simulink library "AvgModels"  (R2015a)
settings: Solver=ode45  StartTime=0.0  StopTime=10.0  RelTol=1e-3
libraries: simulink x12, AvgModels x8
(part 1 of 2)
settings Model: CovSFcnEnable=off  Creator=Luigi Galotto Junior  LastModifiedBy=lgalo
settings DataIOCC: SignalLoggingSaveFormat=ModelDataLogs
settings OptimizationCC: InitFltsAndDblsToZero=on
settings DebuggingCC: SaveWithParameterizedLinksMsg=none  UnderspecifiedInitializationDetection=Classic  MergeDetectMultiDrivingBlocksExec=none  SignalResolutionControl=TryResolveAllWithWarning  SolverPrmCheckMsg=warning  MultiTaskDSMMsg=warning  MultiTaskCondExecSysMsg=none  StrictBusMsg=None
settings GRTTargetCC: TargetFcnLib=ansi_tfl_tmw.mat  CombineOutputUpdateFcns=off  GRTInterface=on

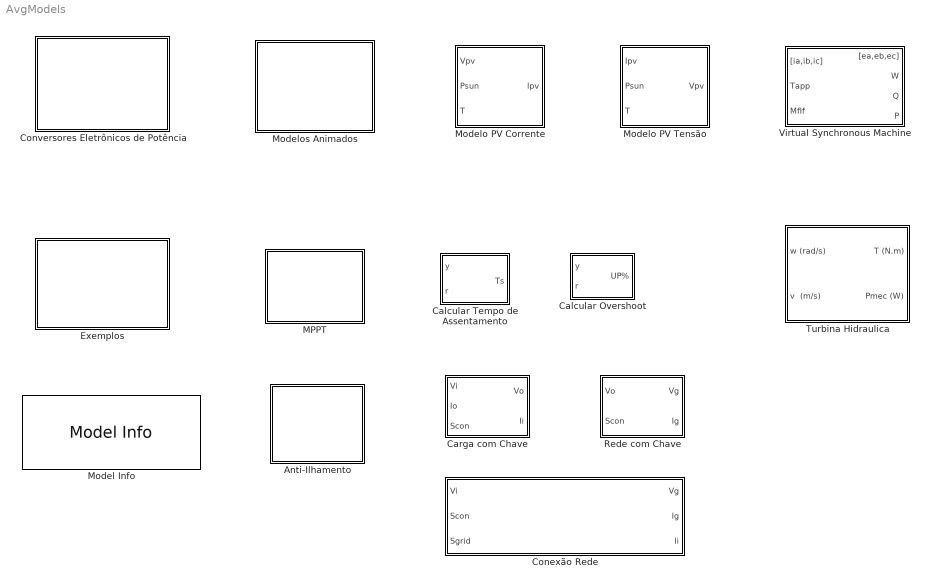
== system AvgModels ==
  Anti-Ilhamento : Subsystem
  Calcular Overshoot : Subsystem  mask(Calc_Up){}
      mask help: Bloco para calcular a Ultrapassagem percentual (UP%) a partir da referência (r) e da resposta da saída (y) no tempo.
  Calcular Tempo de Assentamento : Subsystem  mask(Calc_Ts){}
      mask help: Bloco para calcular o Tempo de Assentamento (Ts), em segundos, a partir da referência (r) e da resposta da saída (y) no tempo.
  Carga com Chave : Subsystem  mask(Modelo Médio de Conexao com a Rede){Rl=100, Rsmin=0.1, Rsmax=1e6}
      mask prompts: Rl "Carga (ohms)"; Rsmin "Resistência on do Relé"; Rsmax "Resistência off do Relé"
      mask help:
      | Simula a conexão de uma fonte de tensão com determinada impedância
      | em uma rede elétrica.
      mask Display:
      | theta = 0:0.1:2*pi;
      | % fundo
      | patch([-1.2 0.3 0.3 -1.2],[-0.1 -0.1 1 1],[1 1 1])
      | 
      | % ------------- circuito da conexao  --------------
      | % circuito
      | plot([-0.9 -0.9 -0.4],[0.1 0.9 0.9])
      | plot([-0.4 -0.3],[0.9 1]) % chave
      | plot([-0.25 0 0],[0.9 0.9 0.1])
      | 
      | % fonte
      | x = 0.15*cos(theta)-0.9;
      | y = 0.15*sin(theta)+0.5;
      | patch(x,y,[1 0.5 0.5]);
      | text(-0.95,0.5,'Vi')
      | 
      | % carga
      | patch([-0.1 0.1 0.1 -0.1],[0.3 0.3 0.6 0.6],[0.5 0.5 1])
      | text(-0.1,0.45,'Rl')
      | 
      | % GND
      | plot([0.80 1]-0.9,[0.1 0.1])
      | plot([0.84 0.96]-0.9,[0.05 0.05])
      | plot([0.88 0.92]-0.9,[0 0]);
      | 
      | plot([0.80 1]-1.8,[0.1 0.1])
      | plot([0.84 0.96]-1.8,[0.05 0.05])
      | plot([0.88 0.92]-1.8,[0 0]);
      | 
      | 
      | % portas
      | port_label('input',1,'Vi')
      | port_label('input',2,'Io')
      | port_label('input',3,'Scon')
      | 
      | port_label('output',1,'Vo')
      | port_label('output',2,'Ii')
  Conexão Rede : Subsystem  mask(Modelo Médio de Conexao com a Rede){Lg=1e-3, Rg=1e-3, Vrede=127, frede=60, Rl=100, Rsmin=0.1, Rsmax=1e6}
      mask prompts: Lg "Indutância da Rede (H)"; Rg "Resistência da Rede (Ohms)"; Vrede "Tensão eficaz da Rede (V)"; frede "Frequência da Rede (Hz)"; Rl "Carga na Rede"; Rsmin "Resistência on do Relé"; Rsmax "Resistência off do Relé"
      mask help:
      | Simula a conexão de uma fonte de tensão com determinada impedância
      | em uma rede elétrica.
      mask Display:
      | theta = 0:0.1:2*pi;
      | % fundo
      | patch([-1.3 1.3 1.3 -1.3],[-0.1 -0.1 1 1],[1 1 1])
      | 
      | % ------------- circuito da conexao  --------------
      | % circuito
      | plot([-0.9 -0.9 -0.4],[0.1 0.9 0.9])
      | plot([-0.4 -0.3],[0.9 1]) % chave
      | plot([-0.25 0 0],[0.9 0.9 0.1])
      | 
      | % fonte
      | x = 0.15*cos(theta)-0.9;
      | y = 0.15*sin(theta)+0.5;
      | patch(x,y,[1 0.5 0.5]);
      | text(-0.95,0.5,'Vi')
      | 
      | % carga
      | patch([-0.1 0.1 0.1 -0.1],[0.3 0.3 0.6 0.6],[0.5 0.5 1])
      | text(-0.05,0.45,'Rl')
      | 
      | % GND
      | plot([0.80 1]-0.9,[0.1 0.1])
      | plot([0.84 0.96]-0.9,[0.05 0.05])
      | plot([0.88 0.92]-0.9,[0 0]);
      | 
      | plot([0.80 1]-1.8,[0.1 0.1])
      | plot([0.84 0.96]-1.8,[0.05 0.05])
      | plot([0.88 0.92]-1.8,[0 0]);
      | 
      | % --------------- circuito da rede -------------
      | % circuito
      | plot([0 0.25],[0.9 0.9])
      | plot([0.3 0.4 0.9 0.9],[1 0.9 0.9 0.1])
      | 
      | % GND
      | plot([0.80 1],[0.1 0.1])
      | plot([0.84 0.96],[0.05 0.05])
      | plot([0.88 0.92],[0 0]);
      | 
      | % controle da chave
      | % plot([0 0.28 0.28],[0.2 0.2 0.9]);
      | 
      | % rede
      | x = 0.15*cos(theta)+0.9;
      | y = 0.15*sin(theta)+0.5;
      | patch(x,y,[1 0.5 0.5])
      | text(0.85,0.5,'Vg')
      | 
      | patch([0.5 0.8 0.8 0.5],[0.8 0.8 1 1],[0.5 0.5 1])
      | text(0.55,0.9,'Zg')
      | 
      | % Texto das chaves
      | text(-0.4,0.7,'Scon')
      | text(0.2,0.7,'Sgrid')
      | 
      | port_label('output',1,'Vg');
      | port_label('output',2,'Ig');
      | port_label('output',2,'Ii');
      | 
      | port_label('input',1,'Vi');
      | port_label('input',2,'Scon');
      | port_label('input',3,'Sgrid');
  Conversores Eletrônicos de Potência : Subsystem
  Exemplos : Subsystem
  MPPT : Subsystem
  Model Info : simulink/Model-Wide Utilities/Model Info  Frame=on  DisplayStringWithTags=|  HorizontalTextAlignment=Center  LeftAlignmentValue=0.5  SourceBlockDiagram=AvgModels  TagMaxNumber=20
      | Conjunto de Blocos de 
      | Modelos Dinâmicos.
      | %<Creator>
      | %<Created>
  Modelo PV Corrente : Subsystem  mask(Modelo PV de corrente){Ms=1, Mp=1, Ns=54, Voc=0.6093, Isc=8.21, Tr=273 + 25, tau=1e-2, Rs=0.005, Rp=7, a=3.18e-3, n=1.2, k=1.38e-23, q=1.60e-19, EG=1.1}
      mask prompts: Ms "Módulos em Série"; Mp "Módulos em Paralelo"; Ns "Número de células"; Voc "Tensão de circuito aberto (Voc por célula)"; Isc "Corrente de curto-circuito (Isc)"; Tr "Temperatura Ambiente (K)"; tau "Constante de Tempo (s)"; Rs "Resistência série"; Rp "Resistência paralela"
      mask help:
      | Este é um modelo de corrente para painéis fotovoltaicos (sozinhos ou em arranjo).
      |
      | Fornece a corrrente esperada de acordo com a tensão, a densidade de potência do sol e a temperatura ambiente.
      |
      | V(PV) é a tensão do arranjo fotovoltaico em volts.
      | Psun é a densidade de potência do sol em W/m2.
      | T é a temperatura ambiente em ºC.
      mask Display:
      | % desenho detalhado
      | patch([0 .5 1 .5],[0 1 1 0],[0 0 1]);
      | plot([0 0.5],[0 1])
      | plot([0.5/3 0.5+0.5/3],[0 1])
      | plot([0.5/3 0.5+0.5/3]+0.5/3,[0 1])
      | plot([0.5 1],[0 1])
      | 
      | plot([0 0.5],[0 0])
      | plot([0 0.5]+0.125,[0 0]+0.25)
      | plot([0 0.5]+0.25,[0 0]+0.5)
      | plot([0 0.5]+0.25+0.125,[0 0]+0.75)
      | plot([0.5 1],[1 1])
      | 
      | 
      | port_label('output',1,'I(PV)');
      | 
      | port_label('input',1,'V(PV)');
      | port_label('input',2,'Psun');
      | port_label('input',3,'T');
  Modelo PV Tensão : Subsystem  mask(Modelo PV de tensão){Ns=54, Voc=0.6093, Isc=8.21, Rs=0.005, Rp=7, Ms=1, Mp=1, Tr=273 + 25, a=3.18e-3, n=1.2, k=1.38e-23, q=1.60e-19, EG=1.1, tau=1e-2, Psun=1000, Animar=on}
      mask prompts: Ns "Número de células"; Voc "Tensão de circuito aberto (Voc por célula)"; Isc "Corrente de curto-circuito (Isc)"; Rs "Resistência série da célula"; Rp "Resistência paralela da célula"; Ms "Módulos em Série"; Mp "Módulos em Paralelo"; Tr "Temperatura Ambiente (K)"; a "Coeficiente de temperatura de Isc:"; n "Fator de qualidade da junção p-n:"; k "Constante de Boltzmann:"; q "Carga do elétron:"; EG "Energia da banda proibida:"; tau "Contante de tempo (s):"; Psun "Irradiação de teste (W/m2):"; Animar "Animar em execução?"
      mask help:
      | Este é um modelo de tensão para painéis fotovoltaicos (sozinhos ou em arranjo).
      |
      | Fornece a tensão esperada de acordo com a corrente, a densidade de potência do sol e a temperatura ambiente.
      |
      | I(PV) é a corrente do arranjo fotovoltaico em Amperes.
      | Psun é a densidade de potência do sol em W/m2.
      | T é a temperatura ambiente em ºC.
      |
      | V(PV) é a tensão do arranjo fotovoltaico em Amperes.
      mask DialogControl Container9 Prompt: Verificação da curva.
      mask DialogControl Control2 Prompt: Verificar Curvas
      mask DialogControl Control2 Callback:
      | Psun = str2num(get_param(gcbh,'Psun'));
      | Tr = str2num(get_param(gcbh,'Tr'));
      | Voc = str2num(get_param(gcbh,'Voc'));
      | Isc = str2num(get_param(gcbh,'Isc'));
      | Rp = str2num(get_param(gcbh,'Rp'));
      | Rs = str2num(get_param(gcbh,'Rs'));
      | Ns = str2num(get_param(gcbh,'Ns'));
      | alpha = str2num(get_param(gcbh,'a'));
      | encontrapmax(Psun,Tr-273,Voc,Isc,Rp,Rs,Ns,alpha);
      mask Display:
      | % desenho detalhado
      | patch([0 .5 1 .5],[0 1 1 0],[0 0 1]);
      | plot([0 0.5],[0 1])
      | plot([0.5/3 0.5+0.5/3],[0 1])
      | plot([0.5/3 0.5+0.5/3]+0.5/3,[0 1])
      | plot([0.5 1],[0 1])
      | 
      | plot([0 0.5],[0 0])
      | plot([0 0.5]+0.125,[0 0]+0.25)
      | plot([0 0.5]+0.25,[0 0]+0.5)
      | plot([0 0.5]+0.25+0.125,[0 0]+0.75)
      | plot([0.5 1],[1 1])
      | 
      | 
      | port_label('output',1,'V(PV)');
      | 
      | port_label('input',1,'I(PV)');
      | port_label('input',2,'Psun');
      | port_label('input',3,'T');
  Modelos Animados : Subsystem
  Rede com Chave : Subsystem  mask(Modelo Médio de Conexao com a Rede){Lg=1e-3, Rg=1e-3, Vrede=127, frede=60, Rsmin=0.1, Rsmax=1e6}
      mask prompts: Lg "Indutância da Rede (H)"; Rg "Resistência da Rede (Ohms)"; Vrede "Tensão eficaz da Rede (V)"; frede "Frequência da Rede (Hz)"; Rsmin "Resistência on do Relé"; Rsmax "Resistência off do Relé"
      mask help:
      | Simula a conexão de uma fonte de tensão em uma rede elétrica
      | com determinada impedância.
      mask Display:
      | theta = 0:0.1:2*pi;
      | % fundo
      | patch([-0.3 1.3 1.3 -0.3],[-0.1 -0.1 1 1],[1 1 1])
      | 
      | % --------------- circuito da rede -------------
      | % circuito
      | plot([0 0.25],[0.9 0.9])
      | plot([0.3 0.4 0.9 0.9],[1 0.9 0.9 0.1])
      | 
      | % GND
      | plot([0.80 1],[0.1 0.1])
      | plot([0.84 0.96],[0.05 0.05])
      | plot([0.88 0.92],[0 0]);
      | 
      | % controle da chave
      | % plot([0 0.28 0.28],[0.2 0.2 0.9]);
      | 
      | % rede
      | x = 0.15*cos(theta)+0.9;
      | y = 0.15*sin(theta)+0.5;
      | patch(x,y,[1 0.5 0.5])
      | text(0.85,0.5,'Vg')
      | 
      | patch([0.5 0.8 0.8 0.5],[0.8 0.8 1 1],[0.5 0.5 1])
      | text(0.55,0.9,'Zg')
      | 
      | 
      | port_label('output',1,'Vg');
      | port_label('output',2,'Ig');
      | 
      | port_label('input',1,'Vi');
      | port_label('input',2,'Scon');
  Turbina Hidraulica : Subsystem  mask(Turbina Pelton){ro=997, Area_bico=(1/4)*pi*0.012^2, gate=Interno (fixo), abertura=1, raio_turbina=0.105, tipo=Pelton, poly=[-0.3915 -0.669 1.52 0.005209]}
      mask prompts: ro "Densidade do fluido (kg/m3)"; Area_bico "Área de entrada do fluido"; gate "Controle do Gate"; abertura "Abertura do Gate (0 a 1)"; raio_turbina "Raio da Turbina"; tipo "Tipos de Turbinas:"; poly "Curva Cp x lambda (polinomio)"
      mask help:
      | Modelo da turbina Pelton em R.P. desenvolvida inicialmente durante
      | o mestrado do acadêmico Júlio Lescano, a partir de dados de um
      | protótipo e de resultados experimentais.
      mask TypeOptions gate: Interno (fixo) | Externo
      mask Callback gate:
      | gate = get_param(gcbh,'gate');
      | p = Simulink.Mask.get(gcb);
      | a = p.Parameters(4);
      | switch gate
      |     case 'Externo'
      |         % a.set('Enable', 'off');
      |     otherwise
      |         % a.set('Enable', 'true');
      | 
      | end
      mask TypeOptions tipo: Pelton | Savonius | Savonius com duto
      mask Callback tipo:
      | tipo = get_param(gcbh,'tipo');
      | switch tipo
      |     case 'Pelton'
      |         set_param(gcbh,'poly','[-0.3915 -0.669 1.52 0.005209]');
      |     case 'Savonius'
      |         set_param(gcbh,'poly','[-0.8682    1.3133   -0.3584]');
      |     case 'Savonius com duto'
      |         set_param(gcbh,'poly','[-0.8682    1.2786   -0.2225]');
      | end
      mask DialogControl Control2 Prompt: Plotar Curvas
      mask DialogControl Control2 Callback:
      | poly = str2num(get_param(gcbh,'poly'));
      | tsr = linspace(0,2,50);
      | plot(tsr,max(polyval(poly,tsr),0))
      | grid;
      | xlabel('\lambda (TSR - Tip Speed Ratio)')
      | ylabel('C_p')
  Virtual Synchronous Machine : Subsystem  mask(Virtual Synchronous Machine (VSM)){J=1e-2, Dpm=1e-4, w0=0}
      mask prompts: J "Inércia:"; Dpm "Atrito Dinâmico:"; w0 "Velocidade Inicial:"
      mask help:
      | Modelo de máquina síncrona virtual (VSM) desenvolvido durante o trabalho de conclusão de curso da aluna Isabela Assis.
      |
      | Objetivo inicial: controlar um inversor emulando uma máquina síncrona, chamado de synchronverter.
      |
      | Também pode ser utilizado como modelo simplificado de máquinas síncronas.

== system AvgModels/Anti-Ilhamento ==
  anti-islanding AFD : Subsystem  mask(Anti-ilhamento AFD){ffalha=62, Df=10}
      mask prompts: ffalha "Frequência de Falha (Hz)"; Df "Variação de frequência (Hz)"
      mask help:
      | Bloco que realiza método ativo de anti-ilhamento AFD (Active Frequency Drift).
      |
      | Pode ser utilizado em conjunto com PLL.
  anti-islanding HF impedance : Subsystem  mask(Anti-ilhamento impedância.){vsinal=2, fsinal=600, vmax=350}
      mask prompts: vsinal "Tensão do Sinal (V)"; fsinal "Frequência do Sinal (Hz)"; vmax "Tensão máxima de detecção (V)"
      mask help:
      | Bloco que realiza método ativo de anti-ilhamento de impedância em alta frequência.
      |
      | Pode ser utilizado em conjunto com PLL.
  anti-islanding SMS : Subsystem  mask(Anti-Ilhamento SMS){fnom=60, fmax=63, angmax=10}
      mask prompts: fnom "Frequência Nominal (Hz)"; fmax "Frequência Máxima (Hz)"; angmax "Ângulo Máximo (graus)"
      mask help:
      | Bloco que realiza método ativo de anti-ilhamento SMS (Sliding Mode Frequency Shift).
      |
      | Pode ser utilizado em conjunto com PLL.

== system AvgModels/Calcular Overshoot ==
  y : Inport
  r : Inport  Port=2
  Difference : simulink/Discrete/Difference  ICPrevInput=0.0  InputProcessing=Inherited  OutMin=[]  OutMax=[]  OutDataType=fixdt(1, 16)  OutScaling=2^-10  DoSatur=off
  Divide : Product  Inputs=*/
  Gain1 : Gain  Gain=100
  Memory : Memory
  Memory1 : Memory
  MinMax : MinMax  Function=max
  MinMax2 : MinMax  Function=max
  Mux1 : Mux  Inputs=2
  Mux2 : Mux  Inputs=2
  Subtract : Sum  Inputs=+-
  amplitude : Display
  UP% : Outport
  wires:
  Memory/1 -> Mux1/2
  Subtract/1 -> Mux1/1
  y/1 -> Subtract/1
  Gain1/1 -> UP%/1
  MinMax/1 -> Divide/1, Memory/1
  Mux1/1 -> MinMax/1
  r/1 -> Difference/1
  Divide/1 -> Gain1/1
  MinMax2/1 -> Memory1/1, amplitude/1, Subtract/2, Divide/2
  Memory1/1 -> Mux2/2
  Difference/1 -> Mux2/1
  Mux2/1 -> MinMax2/1

== system AvgModels/Calcular Tempo de Assentamento ==
  y : Inport
  r : Inport  Port=2
  Abs : Abs
  Compare To Constant : simulink/Logic and Bit Operations/Compare To Constant  relop=>=  const=0.01  OutDataTypeStr=boolean
  Compare To Constant1 : simulink/Logic and Bit Operations/Compare To Constant  relop=>=  const=0.01  OutDataTypeStr=boolean
  Data Type Conversion : DataTypeConversion
  Integrator Limited : Integrator  ExternalReset=falling  LimitOutput=on  LowerSaturationLimit=0
  Logical Operator : Logic  AllPortsSameDT=off
  Sum1 : Sum  Inputs=|+-
  Ts : Outport
  wires:
  Sum1/1 -> Abs/1
  y/1 -> Compare To Constant/1, Integrator Limited/2, Sum1/1
  Integrator Limited/1 -> Ts/1
  Compare To Constant/1 -> Logical Operator/2
  r/1 -> Sum1/2
  Compare To Constant1/1 -> Logical Operator/1
  Data Type Conversion/1 -> Integrator Limited/1
  Abs/1 -> Compare To Constant1/1
  Logical Operator/1 -> Data Type Conversion/1

== system AvgModels/Carga com Chave ==
  Vi : Inport
  Io : Inport  Port=2
  Scon : Inport  Port=3
  Add1 : Sum  Inputs=|+-
  Add2 : Sum  Inputs=|++
  Add3 : Sum  Inputs=|++
  Constant : Constant  Value=Rl
  Product : Product  Inputs=**/
  Product1 : Product
  Product2 : Product  Inputs=*/
  Relay : Relay  OnSwitchValue=0.6  OffSwitchValue=0.4  OnOutputValue=Rsmin  OffOutputValue=Rsmax
  Vo : Outport
  Ii : Outport  Port=2
  wires:
  Product/1 -> Product2/1, Vo/1
  Add2/1 -> Product/3
  Relay/1 -> Add2/2, Product1/2
  Constant/1 -> Product2/2, Product/2, Add2/1
  Scon/1 -> Relay/1
  Vi/1 -> Add1/1
  Io/1 -> Product1/1, Add3/2
  Product1/1 -> Add1/2
  Add1/1 -> Product/1
  Product2/1 -> Add3/1
  Add3/1 -> Ii/1

== system AvgModels/Conexão Rede ==
  Vi : Inport
  Scon : Inport  Port=2
  Sgrid : Inport  Port=3
  Carga com Chave : AvgModels/Carga com Chave  Rl=Rl  Rsmin=Rsmin  Rsmax=Rsmax
  Rede com Chave : AvgModels/Rede com Chave  Lg=Lg  Rg=Rg  Vrede=Vrede  frede=frede  Rsmin=Rsmin  Rsmax=Rsmax
  Vg : Outport
  Ig : Outport  Port=2
  Ii : Outport  Port=3
  wires:
  Carga com Chave/1 -> Rede com Chave/1
  Rede com Chave/1 -> Vg/1
  Rede com Chave/2 -> Carga com Chave/2, Ig/1
  Carga com Chave/2 -> Ii/1
  Vi/1 -> Carga com Chave/1
  Scon/1 -> Carga com Chave/3
  Sgrid/1 -> Rede com Chave/2

== system AvgModels/Conversores Eletrônicos de Potência ==
  Boost : Subsystem  mask(Boost){L=1e-4, RL=0, C=1e-3, Edit_carga=100, Vini=0, Iini=0, Fs=20000, Vdon=0.7, Rdon=0, Vson=0, Rdson=0}
      mask prompts: L "Indutância (H):"; RL "Resistência do Indutor (Ohms):"; C "Capacitância (F):"; Edit_carga "Carga no Capacitor (Ohms):"; Vini "Tensão do Capacitor (V):"; Iini "Corrente do Indutor (A):"; Fs "Frequência de Chaveamento (Hz)"; Vdon "Tensão direta no diodo (V)"; Rdon "Resistência Interna no Diodo"; Vson "Tensão direta na chave (V)"; Rdson "Resistência da Chave"
      mask help:
      | Este bloco modela o comportamento dinâmico médio do conversor CC/CC boost.
      |
      | Este modelo é valido para os modos de condução contínua e descontínua.
      |
      | Quando escolhida a opção (Carga Fixa) a entrada I_out não é utilizada.
      |
      | Desenvolvido por:
      | Luigi Galotto Junior - 21/10/2004
      | Melhorado em 28/09/2017
      mask Display:
      | %image(imread('Boost.jpg'));
      | 
      | % desenho basico
      | %plot([0 1],[0 1])
      | %text(0.3,0.6,'DC')
      | %text(0.6,0.4,'DC')
      | 
      | % desenho detalhado
      | plot([0.0 0.6 0.60 0.5],...
      |      [0.9 0.9 0.60 0.4]);
      | 
      | plot([0 0.6 0.6 0.6 1.1 0.8 0.8 1.1],...
      |      [0 0.0 0.3 0.0 0 0.0 0.9 0.9]);
      | 
      | plot([0.6 0.65 0.65 0.75 0.75 0.75 0.8],...
      |      [0.9 0.90 1.00 0.90 1.00 0.90 0.9])
      | plot([0.6 0.65 0.65 0.75 0.75 0.75 0.8],...
      |      [0.9 0.90 0.80 0.90 0.80 0.90 0.9])
      | 
      | patch([0.25 .5 .5 .25],[0.8 0.8 0.95 0.95],[0 0 1]);
      | patch([0.75 .85 .85 .75],[0.32 0.32 0.6 0.6],[1 0 0]);
      | 
      | text(0.35,0.65,'RL')
      | text(0.65,0.45,'C')
      | 
      | 
      | port_label('output',1,'I in');
      | port_label('output',2,'V out');
      | port_label('input',1,'V in');
      | port_label('input',2,'I out');
      | port_label('input',3,'D');
  Buck : Subsystem  mask(Buck){C=1e-3, L=1e-4, RL=0, Edit_carga=100, Vini=0, Iini=0, Fs=20000, Rdson=10e-3, Vson=0, Rdon=1e-3, Vdon=0.8}
      mask prompts: C "Capacitância (F):"; L "Indutância (H):"; RL "Resistência no Indutor (Ohms):"; Edit_carga "Carga no Capacitor (Ohms)"; Vini "Tensão Inicial do Capacitor (V):"; Iini "Corrente Inicial do Indutor (A):"; Fs "Frequência de Chaveamento (Hz)"; Rdson "Chave (R On)"; Vson "Chave (V On)"; Rdon "Diodo (R On)"; Vdon "Diodo (V On)"
      mask help:
      | Este bloco modela o comportamento dinâmico médio do conversor BUCK CC/CC.
      |
      | Este modelo é valido para os modos de condução contínua e descontínua.
      |
      | Quando escolhida a opção (Carga Fixa) a entrada I_out não é utilizada.
      |
      | Desenvolvido por:
      | Luigi Galotto Junior - 01/10/2017
      mask Display:
      | %image(imread('Boost.jpg'));
      | 
      | % desenho basico
      | plot([0 1],[0 1])
      | text(0.3,0.6,'DC')
      | text(0.6,0.4,'DC')
      | 
      | % desenho detalhado
      | %plot([0.0 0.6 0.60 0.5],...
      | %     [0.9 0.9 0.60 0.4]);
      | 
      | %plot([0 0.6 0.6 0.6 1.1 0.8 0.8 1.1],...
      | %     [0 0.0 0.3 0.0 0 0.0 0.9 0.9]);
      | 
      | %plot([0.6 0.65 0.65 0.75 0.75 0.75 0.8],...
      | %    [0.9 0.90 1.00 0.90 1.00 0.90 0.9])
      | %plot([0.6 0.65 0.65 0.75 0.75 0.75 0.8],...
      | %     [0.9 0.90 0.80 0.90 0.80 0.90 0.9])
      | 
      | %patch([0.25 .5 .5 .25],[0.8 0.8 0.95 0.95],[0 0 1]);
      | %patch([0.75 .85 .85 .75],[0.32 0.32 0.6 0.6],[1 0 0]);
      | 
      | %text(0.35,0.65,'RL')
      | %text(0.65,0.45,'C')
      | 
      | 
      | port_label('output',1,'I in');
      | port_label('output',2,'V out');
      | port_label('input',1,'V in');
      | port_label('input',2,'I out');
      | port_label('input',3,'D');
  Buck-Boost : Subsystem  mask(Buck-Boost){C=1e-3, L=1e-4, RL=0, Edit_carga=100, Vini=0, Iini=0, Fs=20000, Rdson=0, Vson=0, Rdon=0, Vdon=0.8}
      mask prompts: C "Capacitância (F):"; L "Indutância (H):"; RL "Resistência do Indutor (Ohms):"; Edit_carga "Carga no Capacitor (Ohms):"; Vini "Tensão Inicial do Capacitor (V):"; Iini "Corrente Inicial do Indutor (A):"; Fs "Frequência de Chaveamento (Hz)"; Rdson "Chave (R On):"; Vson "Chave (V On):"; Rdon "Diodo (R On):"; Vdon "Diodo (V On):"
      mask help:
      | Este bloco modela o comportamento dinâmico médio do conversor BUCK-BOOST CC/CC.
      |
      | Este modelo é valido para os modos de condução contínua e descontínua.
      |
      | Quando escolhida a opção (Carga Fixa) a entrada I_out não é utilizada.
      |
      | Desenvolvido por:
      | Luigi Galotto Junior - 01/10/2017
      mask Display:
      | %image(imread('Boost.jpg'));
      | 
      | % desenho basico
      | plot([0 1],[0 1])
      | text(0.3,0.6,'DC')
      | text(0.6,0.4,'DC')
      | 
      | % desenho detalhado
      | %plot([0.0 0.6 0.60 0.5],...
      | %     [0.9 0.9 0.60 0.4]);
      | 
      | %plot([0 0.6 0.6 0.6 1.1 0.8 0.8 1.1],...
      | %     [0 0.0 0.3 0.0 0 0.0 0.9 0.9]);
      | 
      | %plot([0.6 0.65 0.65 0.75 0.75 0.75 0.8],...
      | %    [0.9 0.90 1.00 0.90 1.00 0.90 0.9])
      | %plot([0.6 0.65 0.65 0.75 0.75 0.75 0.8],...
      | %     [0.9 0.90 0.80 0.90 0.80 0.90 0.9])
      | 
      | %patch([0.25 .5 .5 .25],[0.8 0.8 0.95 0.95],[0 0 1]);
      | %patch([0.75 .85 .85 .75],[0.32 0.32 0.6 0.6],[1 0 0]);
      | 
      | %text(0.35,0.65,'RL')
      | %text(0.65,0.45,'C')
      | 
      | 
      | port_label('output',1,'I in');
      | port_label('output',2,'V out');
      | port_label('input',1,'V in');
      | port_label('input',2,'I out');
      | port_label('input',3,'D');
  Inversor Boost TriState : Subsystem  mask(Inversor Boost Tri-State){Lb=10e-6, Co=1e-6, ILb=0, Vco=0}
      mask prompts: Lb "Indutância (H)"; Co "Capacitância (F)"; ILb "Corrente do Indutor"; Vco "Tensão no Capacitor"
      mask help:
      | Modelo médio do Inversor Boost Tri-State Integrado.
      |
      | A polaridade da saída é comandada pelo valor de D2 que pode ser positivo ou negativo. O valor máximo de D2 deve ser limitado a 1-D1.
      mask DialogControl Container3 Prompt: Condições Iniciais
      mask Display:
      | %image(imread('Boost.jpg'));
      | 
      | % desenho basico
      | plot([0 1],[0 1])
      | text(0.3,0.6,'DC')
      | text(0.6,0.4,'AC')
      | 
      | % desenho detalhado
      | %plot([0.0 0.6 0.60 0.5],...
      | %     [0.9 0.9 0.60 0.4]);
      | 
      | %plot([0 0.6 0.6 0.6 1.1 0.8 0.8 1.1],...
      | %     [0 0.0 0.3 0.0 0 0.0 0.9 0.9]);
      | 
      | %plot([0.6 0.65 0.65 0.75 0.75 0.75 0.8],...
      | %    [0.9 0.90 1.00 0.90 1.00 0.90 0.9])
      | %plot([0.6 0.65 0.65 0.75 0.75 0.75 0.8],...
      | %     [0.9 0.90 0.80 0.90 0.80 0.90 0.9])
      | 
      | %patch([0.25 .5 .5 .25],[0.8 0.8 0.95 0.95],[0 0 1]);
      | %patch([0.75 .85 .85 .75],[0.32 0.32 0.6 0.6],[1 0 0]);
      | 
      | %text(0.35,0.65,'RL')
      | %text(0.65,0.45,'C')
      | 
      | 
      | port_label('output',1,'I in');
      | port_label('output',2,'V out');
      | port_label('output',3,'I Lin');
      | 
      | port_label('input',1,'V in');
      | port_label('input',2,'I out');
      | port_label('input',3,'D1');
      | port_label('input',4,'D2');
  Inversor Buck-Boost TriState : Subsystem  mask(Inversor Buck-Boost Tri-State){Lb=10e-6, Co=1e-6, ILb=0, Vco=0}
      mask prompts: Lb "Indutância (H)"; Co "Capacitância (F)"; ILb "Corrente do Indutor"; Vco "Tensão no Capacitor"
      mask help:
      | Modelo médio do Inversor Buck-Boost Tri-State Integrado.
      |
      | A polaridade da saída é comandada pelo valor de D2 que pode ser positivo ou negativo. O valor máximo de D2 deve ser limitado a 1-D1.
      mask DialogControl Container3 Prompt: Condições Iniciais
      mask Display:
      | %image(imread('Boost.jpg'));
      | 
      | % desenho basico
      | plot([0 1],[0 1])
      | text(0.3,0.6,'DC')
      | text(0.6,0.4,'AC')
      | 
      | % desenho detalhado
      | %plot([0.0 0.6 0.60 0.5],...
      | %     [0.9 0.9 0.60 0.4]);
      | 
      | %plot([0 0.6 0.6 0.6 1.1 0.8 0.8 1.1],...
      | %     [0 0.0 0.3 0.0 0 0.0 0.9 0.9]);
      | 
      | %plot([0.6 0.65 0.65 0.75 0.75 0.75 0.8],...
      | %    [0.9 0.90 1.00 0.90 1.00 0.90 0.9])
      | %plot([0.6 0.65 0.65 0.75 0.75 0.75 0.8],...
      | %     [0.9 0.90 0.80 0.90 0.80 0.90 0.9])
      | 
      | %patch([0.25 .5 .5 .25],[0.8 0.8 0.95 0.95],[0 0 1]);
      | %patch([0.75 .85 .85 .75],[0.32 0.32 0.6 0.6],[1 0 0]);
      | 
      | %text(0.35,0.65,'RL')
      | %text(0.65,0.45,'C')
      | 
      | 
      | port_label('output',1,'I in');
      | port_label('output',2,'V out');
      | port_label('output',3,'I Lin');
      | 
      | port_label('input',1,'V in');
      | port_label('input',2,'I out');
      | port_label('input',3,'D1');
      | port_label('input',4,'D2');
  Inversor VSI : Subsystem  mask(Inversor Fonte de Tensão (VSI)){Lb=10e-6, Rl=0, Co=1e-6, ILb=0, Vco=0}
      mask prompts: Lb "Indutância do Filtro (H)"; Rl "Resistência do Indutor (Ohms)"; Co "Capacitância do Filtro (F)"; ILb "Corrente do Indutor (A)"; Vco "Tensão no Capacitor (V)"
      mask help:
      | Modelo médio do Inversor Fonte de Tensão (VSI).
      |
      | A polaridade da saída é comandada pelo índice de modulação m, que pode ser positivo ou negativo.
      mask Display:
      | % desenho basico
      | %plot([0 1],[0 1])
      | %text(0.3,0.6,'DC')
      | %text(0.6,0.4,'AC')
      | 
      | %%%%  desenho detalhado %%%%
      | % circuito de saida
      | plot([-0.2 1 0.2 0.2 1.0 -0.2],...
      |      [0 0 0.0 0.9 0.9 0.9]);
      | % circuito entrada
      | plot([-1.5 -0.9 -0.9 -1.5],[-.4 -.4 1.4 1.4]);
      | % bloco de VSI
      | plot([-0.9 -0.2 -0.2 -0.9 -0.9],[-1 -1 2 2 -1]);
      | % RL
      | patch([0 .15 .15 0],[0.75 0.75 1 1],[0 0 1]);
      | % C
      | patch([0.15 .25 .25 .15],[0.3 0.3 0.65 0.65],[1 0 0]);
      | 
      | %port_label('output',2,'IL')
      | %port_label('output',1,'Vo')
      | %port_label('output',3,'Ii')
      | %port_label('input',1,'Vi')
      | %port_label('input',2,'m')
      | %port_label('input',3,'Io')
      | 
      | text(0,1.25,'RL')
      | text(-0.1,0.45,'C')
      | text(-0.7,0.5,'VSI')
      | 
      | 
      | port_label('output',1,'I in');
      | port_label('output',2,'V out');
      | port_label('output',3,'I Lin');
      | 
      | port_label('input',1,'V in');
      | port_label('input',2,'I out');
      | port_label('input',3,'m');
  Queda de Tensão Média Chave e Diodo : Subsystem  mask(Calcular Quedas em Chave e Diodo){Rswitch=50e-3, Uswitch=2.5, Rdiode=1e-3, Udiode=0.7, direction=1}
      mask prompts: Rswitch "Chave (Rds On)"; Uswitch "Chave (V On)"; Rdiode "Diodo (R On)"; Udiode "Diodo (V On)"; direction "Direção (1 para Buck ou Buck-Boost; -1 para Boost)"
      mask help: Modelo utilizado para conversores CC/CC.
  Tempo de Condução do Diodo (MCC ou MCD) : Subsystem  mask(Tempo MCC ou MCD){L=1e-3, Fs=20000}
      mask prompts: L "Indutância (H)"; Fs "Frequência de Chaveamento (Hz)"
      mask help:
      | Determina a fração do período D2 onde ocorrerá a condução do diodo.
      |
      | Se D2 < 1-D1 então estará em Modo de Condução Discontínua (MCD)

== system AvgModels/Exemplos ==
  note: Exemplos de animação de modelos físicos
  note: Exemplos com os painéis fotovoltaicos
  note: Exemplos dos conversores eletrônicos de potência
  Exemplo_Antena : ModelReference  Description=Modelo de Teste do Buck-Boost.  SimulationMode=Normal  CopyOfModelName=<Enter Model Name>
      settings: OpenFcn=Exemplo_Antena
  Exemplo_Robo : ModelReference  Description=Modelo de Teste do Buck-Boost.  SimulationMode=Normal  CopyOfModelName=<Enter Model Name>
      settings: OpenFcn=Exemplo_Robo1dof
  Exemplo_Submarino : ModelReference  Description=Modelo de Teste do Buck-Boost.  SimulationMode=Normal  CopyOfModelName=<Enter Model Name>
      settings: OpenFcn=Exemplo_Submarino
  Exemplo_Suspensao : ModelReference  Description=Modelo de Teste do Buck-Boost.  SimulationMode=Normal  CopyOfModelName=<Enter Model Name>
      settings: OpenFcn=Exemplo_Suspensao
  Teste_Boost : ModelReference  Description=Modelo de Teste do Boost  SimulationMode=Normal  CopyOfModelName=<Enter Model Name>
      settings: OpenFcn=Teste_Boost
  Teste_Buck : ModelReference  Description=Modelo de Teste do Buck.  SimulationMode=Normal  CopyOfModelName=<Enter Model Name>
      settings: OpenFcn=Teste_Buck
  Teste_Buck-Boost : ModelReference  Description=Modelo de Teste do Buck-Boost.  SimulationMode=Normal  CopyOfModelName=<Enter Model Name>
      settings: OpenFcn=Teste_BuckBoost
  Teste_ModeloPV_Corrente : ModelReference  Description=Teste do modelo PV de corrente.  SimulationMode=Normal  CopyOfModelName=<Enter Model Name>
      settings: OpenFcn=Teste_ModeloPV_2015a
  Teste_ModeloPV_Tensão : ModelReference  Description=Teste do modelo PV de tensão.  SimulationMode=Normal  CopyOfModelName=<Enter Model Name>
      settings: OpenFcn=Teste_ModeloPVTensao_2015a
  Teste_VSI : ModelReference  Description=Modelo de Teste do Buck-Boost.  SimulationMode=Normal  CopyOfModelName=<Enter Model Name>
      settings: OpenFcn=Teste_VSI

== system AvgModels/MPPT ==
  MPPT Climbing Hill : Subsystem  mask(MPPT Hill Climbing){fb=628, Passo=10, limsup=0.95, liminf=0, Inicial=0}
      mask prompts: fb "Filtro de derivação:"; Passo "Passo de variação"; limsup "Limite superior da saída:"; liminf "Limite inferior da saída:"; Inicial "Valor inicial:"
      mask help:
      | Algoritmo de rastreamento do ponto de máxima potência (MPPT).
      | Princípio da escalada ou Perturbe and Observe (P&O).
  MPPT InC : Subsystem  mask(MPPT InC){fb=628, Passo=10, limsup=0.95, liminf=0}
      mask prompts: fb "Filtro de derivação:"; Passo "Passo de variação"; limsup "Limite superior da saída:"; liminf "Limite inferior da saída:"
      mask help:
      | Algoritmo de rastreamento do ponto de máxima potência (MPPT).
      | Princípio da condutância incremental (InC).
  MPPT Modified Climbing Hill : Subsystem  mask(MPPT Modified Hill Climbing){fb=628, Escala=1, Passomin=0.1, Passomax=10, Inverso=off, limsup=0.95, liminf=0, Inicial=0}
      mask prompts: fb "Filtro de derivação:"; Escala "Escala de variação:"; Passomin "Passo mínimo:"; Passomax "Passo máximo:"; Inverso "Sentido Inverso?"; limsup "Limite superior da saída:"; liminf "Limite inferior da saída:"; Inicial "Condição Inicial:"
      mask help:
      | Algoritmo de rastreamento do ponto de máxima potência (MPPT).
      | Princípio da escalada ou Perturbe and Observe (P&O) modificado (passo variável).
      |
      |
      | Atualizado - LGJ - 05/2021
  MPPT Oscillation : Subsystem  mask(MPPT Oscillation){wbaixa=100, walta=10, K0=0.1, Kp=0.2, Ki=0.2, limsup=0.95, liminf=0}
      mask prompts: wbaixa "Passa-Baixa (rad/s)"; walta "Passa-Alta (rad/s)"; K0 "K0 (referência de rastreamento)"; limsup "Limite Superior da Saída"; liminf "Limite Inferior da Saída"
      mask help:
      | Algoritmo de rastreamento do ponto de máxima potência (MPPT).
      | Método da oscilação do sistema.
  MPPT V constante : Subsystem  mask(MPPT InC){Voc=32.9, Kp=1, Ki=1, limsup=0.95, liminf=0}
      mask prompts: Voc "Tensão de Circuito Aberto (Voc):"; Kp "Ganho proporcional:"; Ki "Ganho Integral:"; limsup "Limite superior da saída:"; liminf "Limite inferior da saída:"
      mask help:
      | Algoritmo de rastreamento do ponto de máxima potência (MPPT).
      | Princípio da tensão constante.
      | Rastreia para operar com 78% da tensão de circuito aberto (Voc).
  MPPT beta : Subsystem  mask(MPPT Beta){betaref=-18.9261, limsup=0.95, liminf=0, Kp=0.05, Ki=0.8}
      mask prompts: betaref "Referência do Beta"; limsup "Limite Superior da Saída"; liminf "Limite Inferior da Saída"
      mask help:
      | Algoritmo de rastreamento do ponto de máxima potência (MPPT).
      | Método Beta.

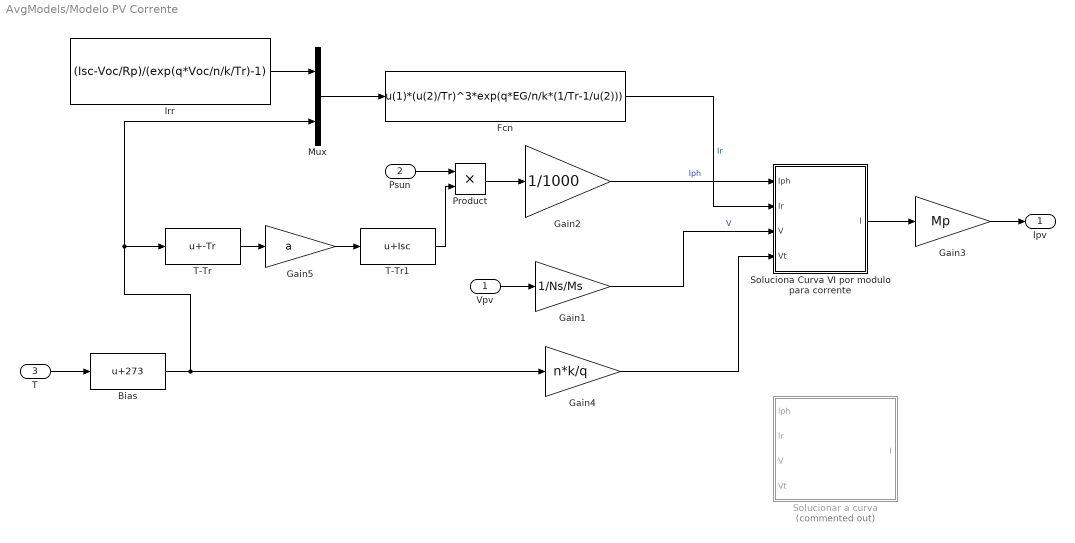
== system AvgModels/Modelo PV Corrente ==
  Vpv : Inport
  Psun : Inport  Port=2
  T : Inport  Port=3
  Bias : Bias  Bias=273
  Fcn : Fcn  Expr=u(1)*(u(2)/Tr)^3*exp(q*EG/n/k*(1/Tr-1/u(2)))
  Gain1 : Gain  Gain=1/Ns/Ms
  Gain2 : Gain  Gain=1/1000
  Gain3 : Gain  Gain=Mp
  Gain4 : Gain  Gain=n*k/q
  Gain5 : Gain  Gain=a
  Irr : Constant  Value=(Isc-Voc/Rp)/(exp(q*Voc/n/k/Tr)-1)
  Mux : Mux  Inputs=2
  Product : Product
  Soluciona Curva VI por modulo para corrente : Subsystem
  Solucionar a curva : Subsystem  Commented=on  TreatAsAtomicUnit=on
  T-Tr : Bias  Bias=-Tr
  T-Tr1 : Bias  Bias=Isc
  Ipv : Outport
  wires:
  Soluciona Curva VI por modulo para corrente/1(I) -> Gain3/1
  Vpv/1 -> Gain1/1
  Gain1/1 -> Soluciona Curva VI por modulo para corrente/3(V)  "V"
  Gain2/1 -> Soluciona Curva VI por modulo para corrente/1(Iph)  "Iph"
  Fcn/1 -> Soluciona Curva VI por modulo para corrente/2(Ir)  "Ir"
  Gain4/1 -> Soluciona Curva VI por modulo para corrente/4(Vt)
  Bias/1 -> Mux/2, T-Tr/1, Gain4/1
  T/1 -> Bias/1
  T-Tr/1 -> Gain5/1
  Gain5/1 -> T-Tr1/1
  Product/1 -> Gain2/1
  T-Tr1/1 -> Product/2
  Psun/1 -> Product/1
  Mux/1 -> Fcn/1
  Irr/1 -> Mux/1
  Gain3/1 -> Ipv/1

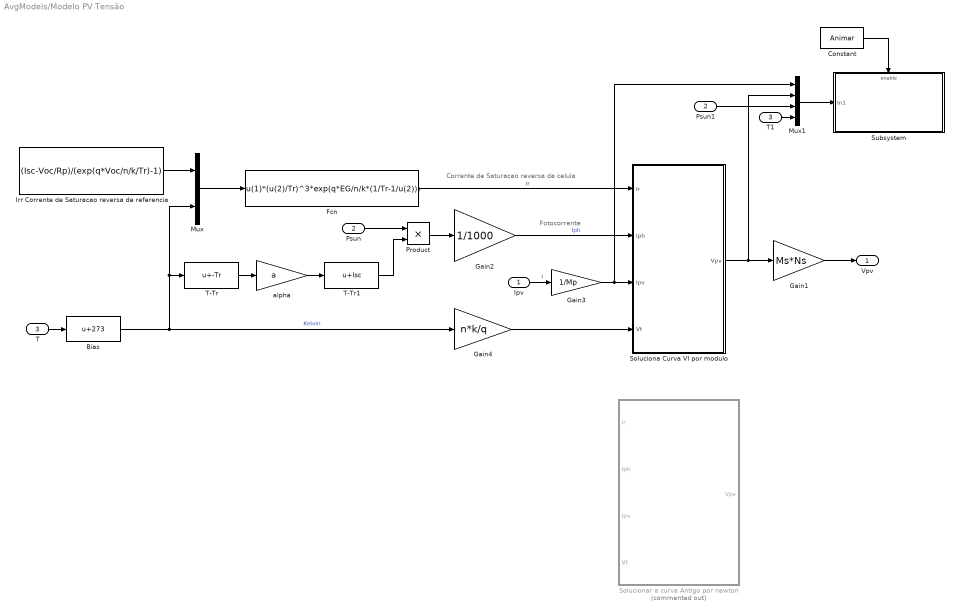
== system AvgModels/Modelo PV Tensão ==
  note: Fotocorrente
  note: Corrente de Saturacao reversa da celula
  Ipv : Inport
  Psun : Inport  Port=2
  T : Inport  Port=3
  Bias : Bias  Bias=273
  Constant : Constant  Value=Animar
  Fcn : Fcn  Expr=u(1)*(u(2)/Tr)^3*exp(q*EG/n/k*(1/Tr-1/u(2)))
  Gain1 : Gain  Gain=Ms*Ns
  Gain2 : Gain  Gain=1/1000
  Gain3 : Gain  Gain=1/Mp
  Gain4 : Gain  Gain=n*k/q
  Irr Corrente de Saturacao reversa de referencia : Constant  Value=(Isc-Voc/Rp)/(exp(q*Voc/n/k/Tr)-1)
  Mux : Mux  Inputs=2
  Mux1 : Mux
  Product : Product
  Psun1 : InportShadow  Port=2
  Soluciona Curva VI por modulo : Subsystem
  Solucionar a curva Antigo por newton : Subsystem  Commented=on  TreatAsAtomicUnit=on
  Subsystem : Subsystem
  T-Tr : Bias  Bias=-Tr
  T-Tr1 : Bias  Bias=Isc
  T1 : InportShadow  Port=3
  alpha : Gain  Gain=a
  Vpv : Outport
  wires:
  Irr Corrente de Saturacao reversa de referencia/1 -> Mux/1
  Mux/1 -> Fcn/1
  Psun/1 -> Product/1
  T-Tr1/1 -> Product/2
  Product/1 -> Gain2/1
  alpha/1 -> T-Tr1/1
  T-Tr/1 -> alpha/1
  T/1 -> Bias/1
  Bias/1 -> T-Tr/1, Mux/2, Gain4/1  "Kelvin"
  Gain4/1 -> Soluciona Curva VI por modulo/4(Vt)
  Fcn/1 -> Soluciona Curva VI por modulo/1(Ir)  "Ir"
  Gain2/1 -> Soluciona Curva VI por modulo/2(Iph)  "Iph"
  Ipv/1 -> Gain3/1  "I"
  Soluciona Curva VI por modulo/1(Vpv) -> Mux1/2, Gain1/1
  Gain1/1 -> Vpv/1
  Gain3/1 -> Mux1/1, Soluciona Curva VI por modulo/3(Ipv)
  Psun1/1 -> Mux1/3
  T1/1 -> Mux1/4
  Mux1/1 -> Subsystem/1(In1)
  Constant/1 -> Subsystem/Enable

== system AvgModels/Modelos Animados ==
  Modelo Antena 1 DOF : Subsystem  mask(Antena){J=1, K=0.1}
      mask prompts: J "Inércia"; K "Ganho"
      mask help:
      | Modelo que reproduz e anima uma antena para ilustração, testes e ensino de sistemas de controle.
      |
      | Considera um sistema de primeira ordem com integrador (tipo 1) para retornar a posição.
  Modelo Braço Robô 1 DOF : Subsystem  mask(BracoRobo){J=1, K=0.1}
      mask prompts: J "Inércia"; K "Ganho"
      mask help:
      | Modelo que reproduz e anima um braço robô para ilustração, testes e ensino de sistemas de controle.
      |
      | Considera um sistema de primeira ordem com integrador (tipo 1) para retornar a posição.
  Submarino Autônomo : Subsystem  mask(Modelo_UFSS){}
      mask help:
      | Simula e anima um submarino autonomo.
      |
      | Retorna a variação da profundidade (h) e o ângulo de inclinação do veículo (Pitch).
      |
      | A entrada (u) é a tensão aplicada no atuador que varia o ângulo do elevador.
  Suspensão 1 DOF : Subsystem  mask(Suspensao_1DOF){M=500, K=10, B=50}
      mask prompts: M "Massa (kg)"; K "Mola (N/m)"; B "Amortecedor (N.s/m)"
      mask help: Modelo de suspensão com (Massa-Mola-Amortecedor) de 2ª ordem, com atuador opcional para suspensão ativa.

== system AvgModels/Rede com Chave ==
  Vo : Inport
  Scon : Inport  Port=2
  Add2 : Sum  Inputs=|++
  Add4 : Sum  Inputs=|+--
  Constant : Constant  Value=Rg
  Gain4 : Gain  Gain=1/Lg
  Integrator : Integrator
  Product : Product
  Rede : Sin  Amplitude=Vrede*sqrt(2)  Frequency=frede*2*pi  SampleTime=0
  Relay : Relay  OnSwitchValue=0.6  OffSwitchValue=0.4  OnOutputValue=Rsmin  OffOutputValue=Rsmax
  Vg : Outport
  Ig : Outport  Port=2
  wires:
  Add4/1 -> Gain4/1
  Rede/1 -> Add4/2, Vg/1  "Vgi"
  Scon/1 -> Relay/1
  Constant/1 -> Add2/1
  Vo/1 -> Add4/1
  Gain4/1 -> Integrator/1
  Integrator/1 -> Ig/1, Product/1
  Relay/1 -> Add2/2
  Add2/1 -> Product/2
  Product/1 -> Add4/3

== system AvgModels/Turbina Hidraulica ==
  w (rad/s) : Inport
  v  (m/s) : Inport  Port=2
  Calculo - Potencia Hidrocinetica : Fcn  Expr=(u(2)*Area_bico*ro*(u(1)^3))/2
  Curva Cp-Lambda : Polyval  Coefs=poly
  Divide : Product  Inputs=*/*
  IC : InitialCondition  Value=0.01
  Lambda CP : simulink/Sinks/XY Graph  Commented=on  xmin=0  xmax=1  ymin=0  ymax=1  st=-1
  Mux : Mux  Inputs=2
  Radius : Constant  Value=raio_turbina
  Saturation : Saturate  UpperLimit=inf  LowerLimit=0
  prod : Product  Inputs=/*
  T (N.m) : Outport
  Pmec (W) : Outport  Port=2
  wires:
  Curva Cp-Lambda/1 -> Lambda CP/2, Mux/2
  Calculo - Potencia Hidrocinetica/1 -> Saturation/1
  Divide/1 -> Lambda CP/1, Curva Cp-Lambda/1
  IC/1 -> prod/1, Divide/1
  Saturation/1 -> Pmec (W)/1, prod/2
  v  (m/s)/1 -> Mux/1, Divide/2
  Radius/1 -> Divide/3
  Mux/1 -> Calculo - Potencia Hidrocinetica/1
  w (rad/s)/1 -> IC/1
  prod/1 -> T (N.m)/1

== system AvgModels/Virtual Synchronous Machine ==
  "[ia,ib,ic]" : Inport
  Tapp : Inport  Port=2
  MfIf : Inport  Port=3
  1/J : Gain  Gain=1/J
  Integrator : Integrator  InitialCondition=w0
  Integrator1 : Integrator  InitialCondition=pi/2
  "Machine Damping Factor " : Gain  Gain=Dpm
  Modelo Elétrico : Subsystem
  Product1 : Product  SaturateOnIntegerOverflow=on  InputSameDT=on  OutDataTypeStr=Inherit: Same as first input
  Sum1 : Sum  Inputs=|+-
  Sum4 : Sum  Inputs=1  SaturateOnIntegerOverflow=on  InputSameDT=on  OutDataTypeStr=Inherit: Same as first input
  Sum5 : Sum  Inputs=-+|
  "[ea,eb,ec]" : Outport
  W : Outport  Port=2
  Q : Outport  Port=3
  P : Outport  Port=4
  wires:
  Product1/1 -> Sum4/1
  Sum4/1 -> P/1
  "[ia,ib,ic]"/1 -> Modelo Elétrico/4(Corrente do Estator [ia,ib,ic]), Product1/1  "Correntes do Estator [ia,ib,ic]"
  Modelo Elétrico/3(Tensão Induzida [ea,eb,ec]) -> "[ea,eb,ec]"/1, Product1/2  "Tensões induzidas [ea,eb,ec]"
  Modelo Elétrico/1(Te) -> Sum1/2  "Te"
  Tapp/1 -> Sum1/1
  Modelo Elétrico/2(Q) -> Q/1  "Output Reactive Power Q"
  "Machine Damping Factor "/1 -> Sum5/1
  Sum5/1 -> 1/J/1
  MfIf/1 -> Modelo Elétrico/3(MfIf)
  1/J/1 -> Integrator/1
  Sum1/1 -> Sum5/2  "Tm - Te"
  Integrator1/1 -> Modelo Elétrico/2(Teta)  "teta"
  Integrator/1 -> "Machine Damping Factor "/1, Integrator1/1, Modelo Elétrico/1(Velocidade Angular do Rotor W), W/1  "W"

== system AvgModels/Anti-Ilhamento/anti-islanding AFD ==
  freal : Inport
  seno real : Inport  Port=2
  + : Sum  Inputs=2
  2*pi : Gain  Gain=2*pi
  Caso de falha : simulink/Logic and Bit Operations/Compare To Constant  relop=>=  const=ffalha  OutDataTypeStr=uint8  ZeroCross=off
  Df : Constant  Value=Df
  Filtro Passa-alta : TransferFcn  Numerator=[1 0]  Denominator=[1/100 1]
  Sat : Saturate  UpperLimit=10e-3  LowerLimit=0
  Sat2 : Saturate  UpperLimit=1000  LowerLimit=0
  Sinal : Signum
  cte : Constant
  rampa com detecção por zero : Integrator  ExternalReset=either
  seno : Trigonometry
  x : Product  RndMeth=Zero
  x2 : Product  RndMeth=Zero
  mod : Outport
  falha : Outport  Port=2
  wires:
  Df/1 -> +/2
  freal/1 -> +/1, Caso de falha/1
  +/1 -> 2*pi/1
  rampa com detecção por zero/1 -> Sat/1
  cte/1 -> rampa com detecção por zero/1
  x/1 -> seno/1
  seno real/1 -> Filtro Passa-alta/1
  seno/1 -> Sat2/1
  Sat2/1 -> x2/1
  x2/1 -> mod/1
  2*pi/1 -> x/1
  Sat/1 -> x/2
  Caso de falha/1 -> falha/1
  Sinal/1 -> x2/2
  Filtro Passa-alta/1 -> Sinal/1, rampa com detecção por zero/2

== system AvgModels/Anti-Ilhamento/anti-islanding HF impedance ==
  Ref. : Inport
  Vo : Inport  Port=2
  + : Sum  Inputs=2
  >= max : simulink/Logic and Bit Operations/Compare To Constant  relop=>=  const=vmax  OutDataTypeStr=uint8  ZeroCross=off
  Abs : Abs
  Sinal de alta frequencia : Sin  Amplitude=vsinal  Frequency=fsinal*2*pi  SampleTime=0
  comparar : Product  RndMeth=Zero
  Ref. modificada : Outport
  falha : Outport  Port=2
  wires:
  Sinal de alta frequencia/1 -> +/2, comparar/1
  Vo/1 -> comparar/2
  Ref./1 -> +/1
  +/1 -> Ref. modificada/1
  comparar/1 -> Abs/1
  Abs/1 -> >= max/1
  >= max/1 -> falha/1

== system AvgModels/Anti-Ilhamento/anti-islanding SMS ==
  freal : Inport
  wt : Inport  Port=2
  Abs : Abs
  Add1 : Sum  Inputs=2
  Add2 : Sum  Inputs=+-
  Add3 : Sum  Inputs=+-
  Divide : Product  Inputs=*/
  ang_max : Gain  Gain=angmax*pi/180
  caso de falha : RelationalOperator  OutDataTypeStr=boolean
  fmax : Constant  Value=fmax
  fnominal : Constant  Value=fnom
  pi/2 : Gain  Gain=pi/2
  seno : Trigonometry
  wt+ang : Outport
  falha : Outport  Port=2
  wires:
  seno/1 -> ang_max/1
  fnominal/1 -> Add2/2, Add3/2
  freal/1 -> Add2/1
  wt/1 -> Add1/1
  Add1/1 -> wt+ang/1
  fmax/1 -> Add3/1
  Add2/1 -> Divide/1, Abs/1
  Add3/1 -> Divide/2, caso de falha/2
  Divide/1 -> pi/2/1
  pi/2/1 -> seno/1
  ang_max/1 -> Add1/2
  Abs/1 -> caso de falha/1
  caso de falha/1 -> falha/1

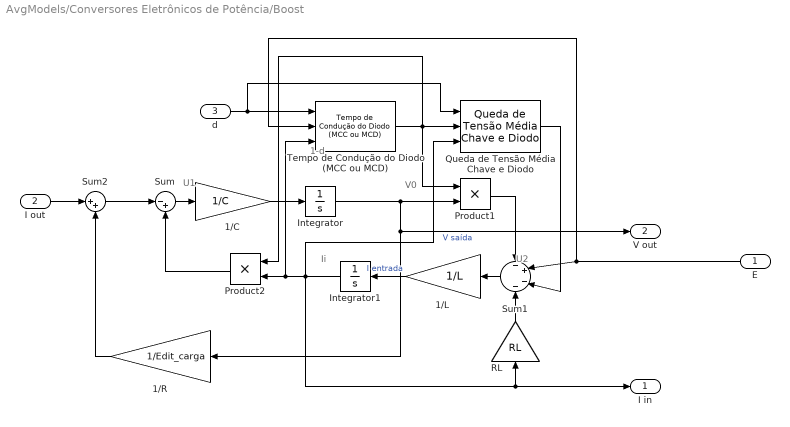
== system AvgModels/Conversores Eletrônicos de Potência/Boost ==
  note: U2
  note: Ii
  note: V0
  note: U1
  note: 1-d
  E : Inport
  I out : Inport  Port=2
  d : Inport  Port=3
  1/C : Gain  Gain=1/C
  1/L : Gain  Gain=1/L
  1/R : Gain  Gain=1/Edit_carga
  Integrator : Integrator  InitialCondition=Vini  LimitOutput=on  LowerSaturationLimit=0
  Integrator1 : Integrator  InitialCondition=Iini  LimitOutput=on  LowerSaturationLimit=0
  Product1 : Product  RndMeth=Zero
  Product2 : Product  RndMeth=Zero
  Queda de Tensão Média Chave e Diodo : AvgModels/Conversores Eletrônicos de Potência/Queda de Tensão Média Chave e Diodo  Rswitch=Rdson  Uswitch=Vson  Rdiode=Rdon  Udiode=Vdon  direction=-1
  RL : Gain  Gain=RL
  Sum : Sum  Inputs=|-+
  Sum1 : Sum  Inputs=-+--
  Sum2 : Sum  Inputs=|++
  Tempo de Condução do Diodo (MCC ou MCD) : AvgModels/Conversores Eletrônicos de Potência/Tempo de Condução  do Diodo (MCC ou MCD)  L=L  Fs=Fs
  I in : Outport
  V out : Outport  Port=2
  wires:
  Integrator1/1 -> Queda de Tensão Média Chave e Diodo/3, Tempo de Condução do Diodo (MCC ou MCD)/3, Product2/2, RL/1, I in/1
  1/C/1 -> Integrator/1
  Product2/1 -> Sum/2
  1/L/1 -> Integrator1/1  "I entrada"
  Sum1/1 -> 1/L/1
  Product1/1 -> Sum1/1
  Integrator/1 -> Product1/2, 1/R/1, V out/1  "V saída"
  Sum/1 -> 1/C/1
  Sum2/1 -> Sum/1
  1/R/1 -> Sum2/2
  E/1 -> Tempo de Condução do Diodo (MCC ou MCD)/2, Sum1/2
  d/1 -> Queda de Tensão Média Chave e Diodo/1, Tempo de Condução do Diodo (MCC ou MCD)/1
  Tempo de Condução do Diodo (MCC ou MCD)/1 -> Queda de Tensão Média Chave e Diodo/2, Product2/1, Product1/1
  I out/1 -> Sum2/1
  Queda de Tensão Média Chave e Diodo/1 -> Sum1/3
  RL/1 -> Sum1/4

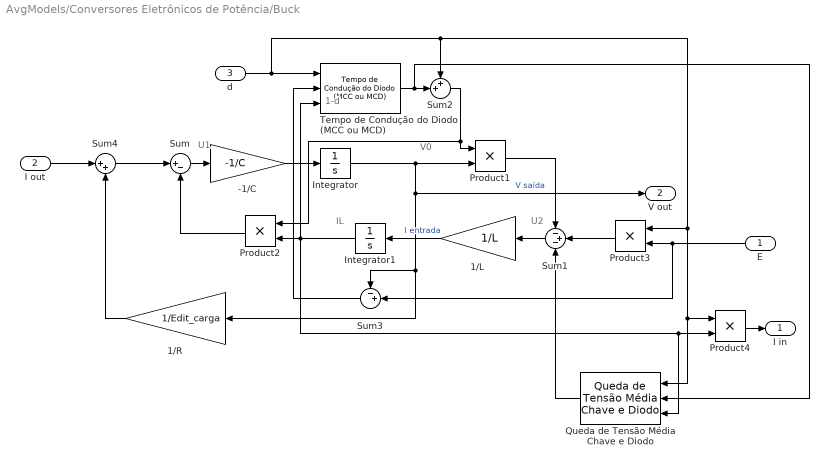
== system AvgModels/Conversores Eletrônicos de Potência/Buck ==
  note: 1-d
  note: U1
  note: V0
  note: IL
  note: U2
  E : Inport
  I out : Inport  Port=2
  d : Inport  Port=3
  -1/C : Gain  Gain=-1/C
  1/L : Gain  Gain=1/L
  1/R : Gain  Gain=1/Edit_carga
  Integrator : Integrator  InitialCondition=Vini  LimitOutput=on  LowerSaturationLimit=0
  Integrator1 : Integrator  InitialCondition=Iini  LimitOutput=on  LowerSaturationLimit=0
  Product{1..4} (4 alike) : Product  RndMeth=Zero
  Queda de Tensão Média Chave e Diodo : AvgModels/Conversores Eletrônicos de Potência/Queda de Tensão Média Chave e Diodo  Rswitch=Rdson  Uswitch=Vson  Rdiode=Rdon  Udiode=Vdon  direction=1
  Sum : Sum  Inputs=|+-
  Sum1 : Sum  Inputs=-+-
  Sum2 : Sum  Inputs=++|
  Sum3 : Sum  Inputs=-+|
  Sum4 : Sum  Inputs=|++
  Tempo de Condução do Diodo (MCC ou MCD) : AvgModels/Conversores Eletrônicos de Potência/Tempo de Condução  do Diodo (MCC ou MCD)  L=L  Fs=Fs
  I in : Outport
  V out : Outport  Port=2
  wires:
  1/R/1 -> Sum4/2
  I out/1 -> Sum4/1
  Sum4/1 -> Sum/1
  Sum/1 -> -1/C/1
  Integrator/1 -> V out/1, Sum3/1, 1/R/1, Product1/2  "V saída"
  Product1/1 -> Sum1/1
  Sum1/1 -> 1/L/1
  1/L/1 -> Integrator1/1  "I entrada"
  Product2/1 -> Sum/2
  -1/C/1 -> Integrator/1
  Integrator1/1 -> Tempo de Condução do Diodo (MCC ou MCD)/3, Queda de Tensão Média Chave e Diodo/3, Product4/2, Product2/2
  Product3/1 -> Sum1/2
  E/1 -> Sum3/2, Product3/2
  Tempo de Condução do Diodo (MCC ou MCD)/1 -> Queda de Tensão Média Chave e Diodo/2, Sum2/2
  d/1 -> Tempo de Condução do Diodo (MCC ou MCD)/1, Sum2/1, Queda de Tensão Média Chave e Diodo/1, Product4/1, Product3/1
  Sum2/1 -> Product2/1, Product1/1
  Product4/1 -> I in/1
  Sum3/1 -> Tempo de Condução do Diodo (MCC ou MCD)/2
  Queda de Tensão Média Chave e Diodo/1 -> Sum1/3

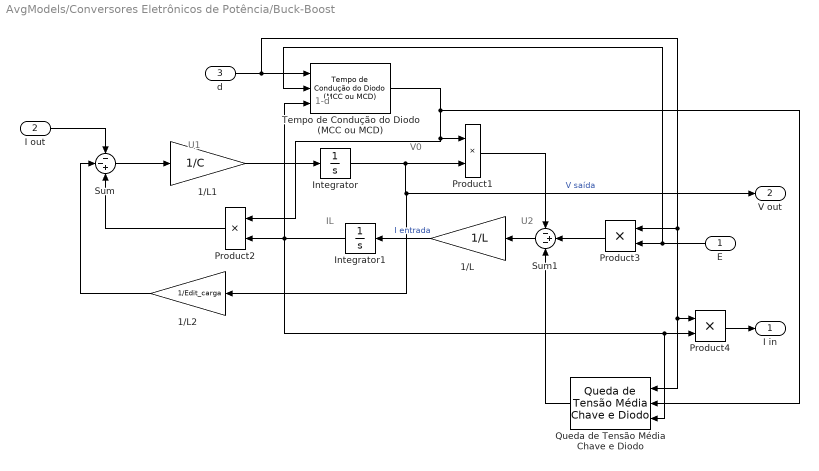
== system AvgModels/Conversores Eletrônicos de Potência/Buck-Boost ==
  note: 1-d
  note: U1
  note: V0
  note: IL
  note: U2
  E : Inport
  I out : Inport  Port=2
  d : Inport  Port=3
  1/L : Gain  Gain=1/L
  1/L1 : Gain  Gain=1/C
  1/L2 : Gain  Gain=1/Edit_carga
  Integrator : Integrator  InitialCondition=Vini  LimitOutput=on  LowerSaturationLimit=0
  Integrator1 : Integrator  InitialCondition=Iini  LimitOutput=on  LowerSaturationLimit=0
  Product{1..4} (4 alike) : Product  RndMeth=Zero
  Queda de Tensão Média Chave e Diodo : AvgModels/Conversores Eletrônicos de Potência/Queda de Tensão Média Chave e Diodo  Rswitch=Rdson  Uswitch=Vson  Rdiode=Rdon  Udiode=Vdon  direction=1
  Sum : Sum  Inputs=--+
  Sum1 : Sum  Inputs=-+-
  Tempo de Condução do Diodo (MCC ou MCD) : AvgModels/Conversores Eletrônicos de Potência/Tempo de Condução  do Diodo (MCC ou MCD)  L=L  Fs=Fs
  I in : Outport
  V out : Outport  Port=2
  wires:
  I out/1 -> Sum/1
  Sum/1 -> 1/L1/1
  Integrator/1 -> 1/L2/1, V out/1, Product1/2  "V saída"
  Product1/1 -> Sum1/1
  Sum1/1 -> 1/L/1
  1/L/1 -> Integrator1/1  "I entrada"
  Product2/1 -> Sum/3
  1/L1/1 -> Integrator/1
  Integrator1/1 -> Tempo de Condução do Diodo (MCC ou MCD)/3, Queda de Tensão Média Chave e Diodo/3, Product4/2, Product2/2
  Product3/1 -> Sum1/2
  d/1 -> Tempo de Condução do Diodo (MCC ou MCD)/1, Queda de Tensão Média Chave e Diodo/1, Product4/1, Product3/1
  Tempo de Condução do Diodo (MCC ou MCD)/1 -> Queda de Tensão Média Chave e Diodo/2, Product2/1, Product1/1
  Product4/1 -> I in/1
  E/1 -> Tempo de Condução do Diodo (MCC ou MCD)/2, Product3/2
  Queda de Tensão Média Chave e Diodo/1 -> Sum1/3
  1/L2/1 -> Sum/2

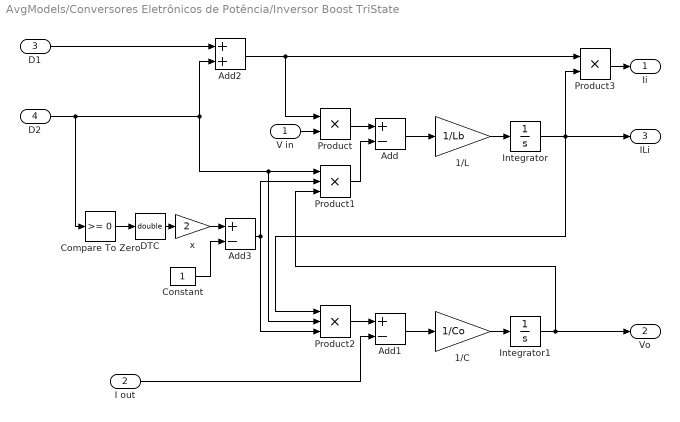
== system AvgModels/Conversores Eletrônicos de Potência/Inversor Boost TriState ==
  V in : Inport
  I out : Inport  Port=2
  D1 : Inport  Port=3
  D2 : Inport  Port=4
  1/C : Gain  Gain=1/Co
  1/L : Gain  Gain=1/Lb
  Add : Sum  Inputs=+-
  Add1 : Sum  Inputs=+-
  Add2 : Sum  Inputs=2
  Add3 : Sum  Inputs=+-
  Compare To Zero : simulink/Logic and Bit Operations/Compare To Zero  relop=>=  OutDataTypeStr=boolean
  Constant : Constant
  DTC : DataTypeConversion  OutDataTypeStr=double
  Integrator : Integrator  InitialCondition=ILb  LimitOutput=on  LowerSaturationLimit=0
  Integrator1 : Integrator  InitialCondition=Vco  LowerSaturationLimit=0
  Product : Product  RndMeth=Zero
  Product1 : Product  Inputs=3  RndMeth=Zero
  Product2 : Product  Inputs=3  RndMeth=Zero
  Product3 : Product  RndMeth=Zero
  x : Gain  Gain=2  OutDataTypeStr=double  RndMeth=Round
  Ii : Outport
  Vo : Outport  Port=2
  ILi : Outport  Port=3
  wires:
  D1/1 -> Add2/1
  V in/1 -> Product/2
  Compare To Zero/1 -> DTC/1
  Product/1 -> Add/1
  Product1/1 -> Add/2
  Add/1 -> 1/L/1
  1/L/1 -> Integrator/1
  Integrator/1 -> ILi/1, Product2/1, Product3/2
  Product2/1 -> Add1/1
  I out/1 -> Add1/2
  1/C/1 -> Integrator1/1
  Add1/1 -> 1/C/1
  Integrator1/1 -> Vo/1, Product1/3
  Product3/1 -> Ii/1
  Add2/1 -> Product/1, Product3/1
  x/1 -> Add3/1
  Add3/1 -> Product1/2, Product2/3
  Constant/1 -> Add3/2
  DTC/1 -> x/1
  D2/1 -> Compare To Zero/1, Product2/2, Product1/1, Add2/2

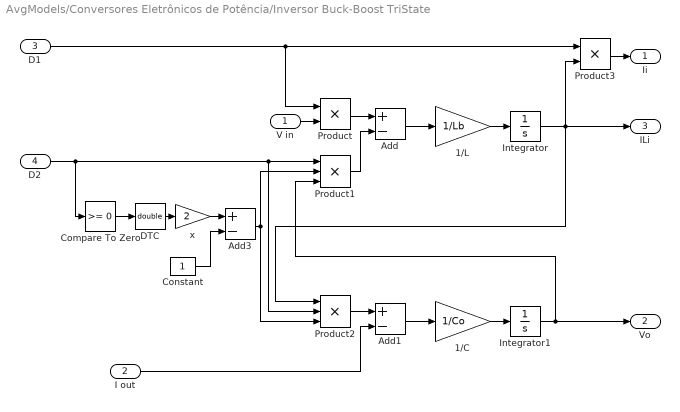
== system AvgModels/Conversores Eletrônicos de Potência/Inversor Buck-Boost TriState ==
  V in : Inport
  I out : Inport  Port=2
  D1 : Inport  Port=3
  D2 : Inport  Port=4
  1/C : Gain  Gain=1/Co
  1/L : Gain  Gain=1/Lb
  Add : Sum  Inputs=+-
  Add1 : Sum  Inputs=+-
  Add3 : Sum  Inputs=+-
  Compare To Zero : simulink/Logic and Bit Operations/Compare To Zero  relop=>=  OutDataTypeStr=boolean
  Constant : Constant
  DTC : DataTypeConversion  OutDataTypeStr=double
  Integrator : Integrator  InitialCondition=ILb  LimitOutput=on  LowerSaturationLimit=0
  Integrator1 : Integrator  InitialCondition=Vco  LowerSaturationLimit=0
  Product : Product  RndMeth=Zero
  Product1 : Product  Inputs=3  RndMeth=Zero
  Product2 : Product  Inputs=3  RndMeth=Zero
  Product3 : Product  RndMeth=Zero
  x : Gain  Gain=2  OutDataTypeStr=double  RndMeth=Round
  Ii : Outport
  Vo : Outport  Port=2
  ILi : Outport  Port=3
  wires:
  D2/1 -> Product1/1, Product2/2, Compare To Zero/1
  DTC/1 -> x/1
  Constant/1 -> Add3/2
  Add3/1 -> Product2/3, Product1/2
  x/1 -> Add3/1
  D1/1 -> Product3/1, Product/1
  Product3/1 -> Ii/1
  Integrator1/1 -> Product1/3, Vo/1
  Add1/1 -> 1/C/1
  1/C/1 -> Integrator1/1
  I out/1 -> Add1/2
  Product2/1 -> Add1/1
  Integrator/1 -> Product3/2, Product2/1, ILi/1
  1/L/1 -> Integrator/1
  Add/1 -> 1/L/1
  Product1/1 -> Add/2
  Product/1 -> Add/1
  Compare To Zero/1 -> DTC/1
  V in/1 -> Product/2
